simulink model "PID_Controller"  (R2020b)
settings: Solver=VariableStepAuto  StartTime=0.0  StopTime=10.0  RelTol=1e-3
values from neighbouring files (symbols this model uses):
  Kd = 0.15    [Dict_Assignment_4.sldd]
  Ki = 500.0    [Dict_Assignment_4.sldd]
  Kp = 21.0    [Dict_Assignment_4.sldd]
settings Model: DataDictionary=Dict_Assignment_4.sldd  Creator=Shantam Garg  LastModifiedBy=Shantam Garg
settings DataIOCC: SaveOutput=off  SaveTime=off

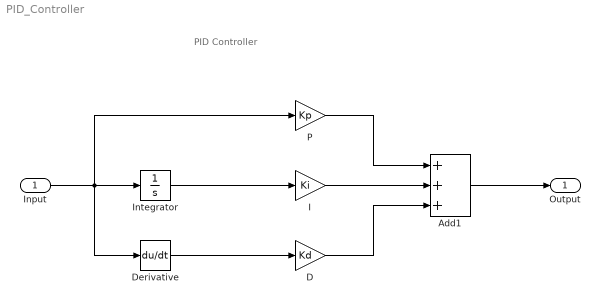
== system PID_Controller ==
  note: PID Controller
  Input : Inport  OutDataTypeStr=double  PortDimensions=1  SampleTime=0
  Add1 : Sum  Inputs=+++
  D : Gain  Gain=Kd
  Derivative : Derivative
  I : Gain  Gain=Ki
  Integrator : Integrator
  P : Gain  Gain=Kp
  Output : Outport  OutDataTypeStr=double  PortDimensions=1  SampleTime=0
  wires:
  P/1 -> Add1/1
  Input/1 -> Integrator/1, Derivative/1, P/1
  Integrator/1 -> I/1
  D/1 -> Add1/3
  Add1/1 -> Output/1
  Derivative/1 -> D/1
  I/1 -> Add1/2
